simulink model "simple"  (R2018a)
settings: Solver=ode5  StartTime=0.0  StopTime=tf  FixedStep=Ts  RelTol=1e-3
model workspace (MAT data in the model file):
  t_sig = mpt.Signal
  t_sig.DataType = 'auto'
  t_sig.Dimensions = -1
  t_sig.DimensionsMode = 'auto'
  t_sig.Complexity = 'auto'
  t_sig.SampleTime = -1
  t_sig.SamplingMode = 'auto'
  u_sig = mpt.Signal
  u_sig.DataType = 'auto'
  u_sig.Dimensions = -1
  u_sig.DimensionsMode = 'auto'
  u_sig.Complexity = 'auto'
  u_sig.SampleTime = -1
  u_sig.SamplingMode = 'auto'
  y_sig = mpt.Signal
  y_sig.DataType = 'auto'
  y_sig.Dimensions = -1
  y_sig.DimensionsMode = 'auto'
  y_sig.Complexity = 'auto'
  y_sig.SampleTime = -1
  y_sig.SamplingMode = 'auto'
values from neighbouring files (symbols this model uses):
  B = mpt.Parameter    [pend_init.m]    (also in test.m)
  g = 9.8    [eml_pend_dyn.m]    (also in pend_init.m = mpt.Parameter; test.m = mpt.Parameter)
  k = mpt.Parameter    [pend_init.m]    (also in test.m)
  l = 1    [eml_pend_dyn.m]    (also in pend_init.m = mpt.Parameter; test.m = mpt.Parameter)
  m = 1    [eml_pend_dyn.m]    (also in pend_init.m = mpt.Parameter; test.m = mpt.Parameter)
  x_ddot_0 = Simulink.Parameter    [pend_init.m]    (also in test.m)
  x_dot_0 = Simulink.Parameter    [pend_init.m]    (also in test.m)
settings Model: Creator=sam  LastModifiedBy=sam
settings OptimizationCC: DefaultParameterBehavior=Inlined  BufferReuse=off  GlobalBufferReuse=off  ExpressionFolding=off  EnableMemcpy=off  PassReuseOutputArgsAs=Individual arguments  LocalBlockOutputs=off  OptimizeDataStoreBuffers=off  BusAssignmentInplaceUpdate=off  OptimizationLevel=level0  OptimizationCustomize=off
settings DebuggingCC: MultiTaskCondExecSysMsg=warning  MultiTaskRateTransMsg=warning  ParameterTunabilityLossMsg=error
settings HardwareCC: TargetBitPerLong=64  TargetBitPerPointer=64  TargetBitPerSizeT=64  TargetBitPerPtrDiffT=64  TargetLongLongMode=on  TargetIntDivRoundTo=Zero  TargetEndianess=LittleEndian  TargetWordSize=64  TargetHWDeviceType=MATLAB Host  ProdEqTarget=off
settings SFSimCC: MATLABDynamicMemAlloc=off
settings RTWCC: SystemTargetFile=ert_shrlib.tlc  TemplateMakefile=ert_default_tmf  Description=Embedded Coder (host-based shared library target)  IncludeHyperlinkInReport=on
settings CodeAppCC: ForceParamTrailComments=on  IgnoreCustomStorageClasses=off  OperatorAnnotations=on  SimulinkDataObjDesc=on  SFDataObjDesc=on  InsertBlockDesc=on
settings STFCustomTargetCC: TargetLangStandard=C99 (ISO)  MultiwordLength=256  GenerateSampleERTMain=on  ParMdlRefBuildCompliant=on  CompOptLevelCompliant=on  CombineOutputUpdateFcns=on  ERTCustomFileBanners=on  SupportComplex=off  SupportNonInlinedSFcns=off  RemoveResetFunc=on  MATLABClassNameForMDSCustomization=Simulink.SoftwareTarget.ERTCustomization  ModelStepFunctionPrototypeControlCompliant=on  GRTInterface=off  UseToolchainInfoCompliant=on  SystemTargetFile=ert_shrlib.tlc
settings ERTTargetCC: TargetLangStandard=C99 (ISO)  GenerateSampleERTMain=on  ConcurrentExecutionCompliant=off  SupportComplex=off  SupportContinuousTime=on  CPPClassGenCompliant=off  InlinedParameterPlacement=NonHierarchical  ERTCustomFileTemplate=example_file_process.tlc

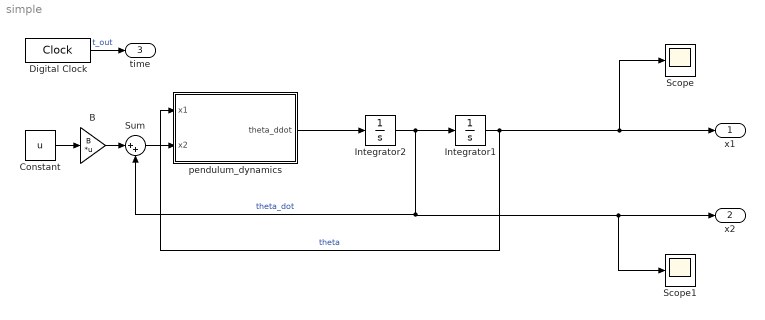
== system simple ==
  B : Gain  Gain=B  Multiplication=Matrix(K*u)
  Constant : Constant  Value=u
  Digital Clock : DigitalClock  SampleTime=1/200
  Integrator1 : Integrator  InitialCondition=x_dot_0
  Integrator2 : Integrator  InitialCondition=x_ddot_0
  Scope : Scope
  Scope1 : Scope
  Sum : Sum  Inputs=|++
  pendulum_dynamics : Subsystem
  x1 : Outport
  x2 : Outport  Port=2
  time : Outport  Port=3
  wires:
  Digital Clock/1 -> time/1  "t_out"
  Constant/1 -> B/1
  B/1 -> Sum/1
  pendulum_dynamics/1(theta_ddot) -> Integrator2/1
  Integrator2/1 -> Scope1/1, x2/1, Sum/2, Integrator1/1  "theta_dot"
  Integrator1/1 -> pendulum_dynamics/1(x1), Scope/1, x1/1  "theta"
  Sum/1 -> pendulum_dynamics/2(x2)

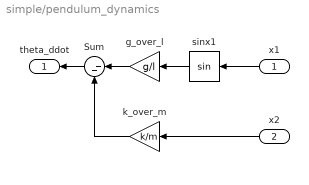
== system simple/pendulum_dynamics ==
  x1 : Inport
  x2 : Inport  Port=2
  Sum : Sum  Inputs=|--
  g_over_l : Gain  Gain=g/l
  k_over_m : Gain  Gain=k/m
  sinx1 : Trigonometry
  theta_ddot : Outport
  wires:
  sinx1/1 -> g_over_l/1
  g_over_l/1 -> Sum/1
  k_over_m/1 -> Sum/2
  x1/1 -> sinx1/1
  x2/1 -> k_over_m/1
  Sum/1 -> theta_ddot/1
